simulink model "Abhi"  (R2025a)
settings: Solver=ode45  StartTime=0.0  StopTime=1  RelTol=1e-3  EnableMultiTasking=on
values from neighbouring files (symbols this model uses):
  Bf = 0.001    [Moedl.m]    (also in srm_mpc_setup.m)
  Bp1_Current = linspace(0,180,181)    [Lut.m]    (also in Lut_1.m; Lut_Model.m)
  Bp2_Current = linspace(0,0.50,101)    [Lut.m]    (also in Lut_1.m = linspace(0,10,101); Lut_Model.m = linspace(0,10,101))
  J = 0.01    [CODE.m]    (also in Controller.m = 0.001; Lut.m; Moedl.m; srm_mpc_setup.m)
  LuT_Current = zeros(length(Bp1_Current), length(Bp2_Current))    [Lut.m]    (also in Lut_1.m; Lut_Model.m = zeros(181,101))
  Rs = 1    [CODE.m]    (also in Moedl.m; srm_mpc_setup.m)
undefined symbols (not defined in the file or in its folder): Ion, Lithium
libraries: spsDiodeLib x8, spsSeriesRLCBranchLib x8, spsIGBTLib x6, spsVoltageMeasurementLib x5, spsCurrentMeasurementLib x4, spsMosfetLib x3, simulink_need_slupdate x2, simulink x2, spsBatteryLib x1, mpclib x1, sps_lib x1, spspowerguiLib x1
settings Model: Creator=user 1  LastModifiedBy=srima
settings SolverCC: AlgebraicLoopSolver=TrustRegion
settings DataIOCC: LimitDataPoints=on  SaveFormat=Array  SignalLoggingSaveFormat=ModelDataLogs  ReturnWorkspaceOutputs=off
settings OptimizationCC: ExpressionDepthLimit=2147483647.0  LifeSpan=inf
settings DebuggingCC: UnderspecifiedInitializationDetection=Classic  MergeDetectMultiDrivingBlocksExec=none  SolverPrmCheckMsg=warning  FcnCallInpInsideContextMsg=warning  UnconnectedInputMsg=warning  UnconnectedOutputMsg=warning  UnconnectedLineMsg=warning  StateNameClashWarn=warning  SFUnexpectedBacktrackingDiag=warning  SFNoUnconditionalDefaultTransitionDiag=warning  SFExecutionAtInitializationDiag=none  ArithmeticOperatorsInVariantConditions=warning
settings HardwareCC: ProdBitPerPointer=32.0  ProdBitPerSizeT=32.0  ProdBitPerPtrDiffT=32.0  ProdLargestAtomicFloat=None  ProdIntDivRoundTo=Undefined  ProdEndianess=Unspecified  ProdWordSize=32.0  ProdHWDeviceType=32-bit Generic
settings ModelReferenceCC: PropagateSignalLabelsOutOfModel=off
settings SFSimCC: SimUseLocalCustomCode=off  CustomCodeUndefinedFunction=UseInterfaceOnly
settings RTWCC: RTWUseLocalCustomCode=off  GPUComputeCapability=3.5
settings CodeAppCC: StateflowObjectComments=on
settings GRTTargetCC: TargetLangStandard=C89/C90 (ANSI)  CombineOutputUpdateFcns=off  GRTInterface=on
settings ConfigComp: CovMetricSettings=dw  CovSaveCumulativeToWorkspaceVar=on  CovSaveSingleToWorkspaceVar=on  CovExternalEMLEnable=off
settings SimscapeCC: SimscapeNormalizeSystem=off
settings ConfigurationSet: Description=SimMechanics 2G

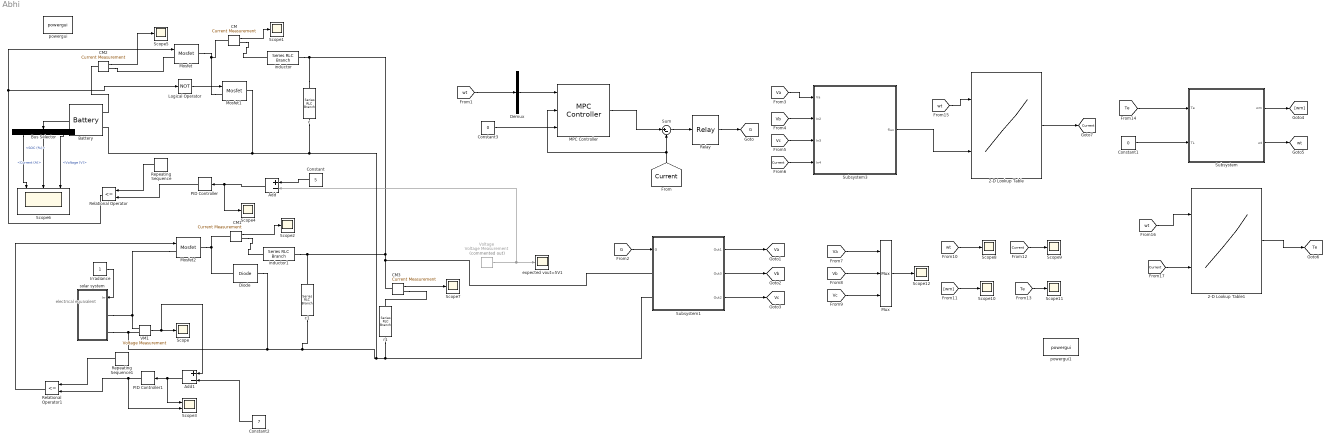
== system Abhi ==
  note: electrical
      | equivalent
  2-D Lookup Table : Lookup_n-D  BreakpointsForDimension1=Bp1_Current  BreakpointsForDimension2=Bp2_Current  Table=LuT_Current  InternalRulePriority=Speed  RndMeth=Simplest
      settings: InputPortMap=u0,u1
  2-D Lookup Table1 : Lookup_n-D  BreakpointsForDimension1=Bp1_Current  BreakpointsForDimension2=Bp2_Current  Table=LuT_Current  InternalRulePriority=Speed  RndMeth=Simplest
      settings: InputPortMap=u0,u1
  Add : Sum  Inputs=+-
  Add1 : Sum  Inputs=+-
  Battery : spsBatteryLib/Battery  BatType=Lithium-Ion  NomV=12  NomQ=6.5  SOC=50  Batt_Tr=30  PresetModel=on  MaxQ=6.5  MinV=9  FullV=13.9678  Dis_rate=2.8261  R=0.018462  Normal_OP=5.8783  expZone="[12.9646     0.319348]"
      settings: LibrarySourceBlock=electricdrivelib/Extra Sources/Battery
  Bus Selector : BusSelector  OutputSignals=SOC (%),Current (A),Voltage (V)
  CM{,1..3} (4 alike) : spsCurrentMeasurementLib/Current Measurement  PhasorSimulation=off  OutputType=Complex  PSBequivalent=0
  Constant : Constant  Value=5
  Constant1 : Constant  Value=0
  Constant2 : Constant  Value=7
  Constant3 : Constant  Value=0
  Demux : Demux  Outputs=3
  Diode : spsDiodeLib/Diode  Ron=0.001  Lon=0  Vf=0.8  IC=0  UseSnubber=off  Rs=500  Cs=250e-9  Measurements=off
  Irradiance : Constant
  Logical Operator : Logic  Operator=NOT  AllPortsSameDT=off  OutDataTypeStr=boolean
  MPC Controller : mpclib/MPC Controller  SCDEnableBlockLinearizationSpecification=on  mpcobj=mpcobj  is_multiple=0  enable_value=0  return_u0=off  updateMPCinCallerWorkspace=on  md_inport=on  mv_inport=off  uref_inport=off  return_cost=off  return_mvseq=off  return_qpstatus=off  return_xseq=off  return_state=off  return_ovseq=off  state_inport=off  umin_inport=off  umax_inport=off  ymin_inport=off  ymax_inport=off  cc_inport=off  ywt_inport=off  uwt_inport=off  duwt_inport=off  rhoeps_inport=off  pm_inport=off  MaximumP=10  HorizonChoice=FixedHorizon  n_ts=0.001  n_p=10  n_mv=1  n_md=1  n_ud=0  n_mo=1  n_uo=0  BlockDataType=double  SampleTimeInherited=off  switch_inport=off
  Mosfet : spsMosfetLib/Mosfet  Ron=0.1  Lon=0  Rd=0.01  Vfd=0  IC=0  Rs=1e5  Cs=inf  Measurements=off
  Mosfet1 : spsMosfetLib/Mosfet  Ron=0.1  Lon=0  Rd=0.01  Vfd=0  IC=0  Rs=1e5  Cs=inf  Measurements=off
  Mosfet2 : spsMosfetLib/Mosfet  Ron=0.1  Lon=0  Rd=0.01  Vfd=0  IC=0  Rs=1e5  Cs=inf  Measurements=off
  Mux : Mux  Inputs=3
  PID Controller : simulink_need_slupdate/PID Controller  P=1  I=5  D=0
  PID Controller1 : simulink_need_slupdate/PID Controller  P=1  I=5  D=0
  Relational Operator : RelationalOperator  Operator=<=  OutDataTypeStr=boolean  InputSameDT=off
  Relational Operator1 : RelationalOperator  Operator=<=  OutDataTypeStr=boolean  InputSameDT=off
  Relay : Relay  OnSwitchValue=10  OffSwitchValue=-10
  Repeating Sequence : simulink/Sources/Repeating Sequence  rep_seq_t=[0 .5/15e3 1/15e3]  rep_seq_y=[0 1 0]
  Repeating Sequence1 : simulink/Sources/Repeating Sequence  rep_seq_t=[0 .5/15e3 1/15e3]  rep_seq_y=[0 1 0]
  Scope{,1..2,4..5,7..12} (11 alike) : Scope
      Scope settings: DataLoggingDecimation=1000  DataLoggingVariableName=pvv  DataLoggingSaveFormat=Array
      Scope1 settings: ActiveDisplayYMinimum=0.5751  ActiveDisplayYMaximum=0.576  DataLoggingDecimation=1000  DataLoggingVariableName=xxbat  DataLoggingSaveFormat=Array
      Scope10 settings: ActiveDisplayYMinimum=-476.34813632584394  ActiveDisplayYMaximum=729.585973445895  DataLoggingVariableName=ScopeData2
      Scope11 settings: ActiveDisplayYMinimum=-0.1626541818945092  ActiveDisplayYMaximum=1.1678030879482377  DataLoggingVariableName=ScopeData5
      Scope12 settings: ActiveDisplayYMinimum=-1  ActiveDisplayYMaximum=1  DataLoggingVariableName=ScopeData6
      Scope2 settings: ActiveDisplayYMinimum=0.5751  ActiveDisplayYMaximum=0.576  DataLoggingDecimation=1000  DataLoggingVariableName=xxpv  DataLoggingSaveFormat=Array
      Scope4 settings: ActiveDisplayYMinimum=-0.7  ActiveDisplayYMaximum=0.5  DataLoggingVariableName=ScopeData3
      Scope5 settings: ActiveDisplayYMinimum=0.5751  ActiveDisplayYMaximum=0.576
      Scope7 settings: ActiveDisplayYMinimum=0.5751  ActiveDisplayYMaximum=0.576  DataLoggingDecimation=1000  DataLoggingVariableName=ioutt  DataLoggingSaveFormat=Array
      Scope8 settings: ActiveDisplayYMinimum=-31.606367633702448  ActiveDisplayYMaximum=124.63641119185642  DataLoggingVariableName=ScopeData8
      Scope9 settings: ActiveDisplayYMinimum=-16.407831336073173  ActiveDisplayYMaximum=26.585137451744139
  Scope3 : Scope  NumInputPorts=2
      settings: ActiveDisplayYMinimum=0.5751  ActiveDisplayYMaximum=0.576  DataLoggingVariableName=ScopeData4
  Scope6 : Scope  NumInputPorts=3
      settings: ActiveDisplayYMinimum=47.5013  ActiveDisplayYMaximum=52.5015  DataLoggingVariableName=ScopeData7
  Subsystem : Subsystem
  Subsystem1 : Subsystem
  Subsystem3 : Subsystem
  Sum : Sum  Inputs=|+-
  VM1 : spsVoltageMeasurementLib/Voltage Measurement  PhasorSimulation=off  OutputType=Complex  PSBequivalent=0
  Voltage : spsVoltageMeasurementLib/Voltage Measurement  Commented=on  PhasorSimulation=off  OutputType=Complex  PSBequivalent=0
  c : spsSeriesRLCBranchLib/Series RLC Branch  LConnTagsString=__new0  RConnTagsString=__new0  BranchType=C  Resistance=1  Inductance=1e-3  SetiL0=off  InitialCurrent=0  Capacitance=160e-6  Setx0=off  InitialVoltage=0  Measurements=None
  c1 : spsSeriesRLCBranchLib/Series RLC Branch  LConnTagsString=__new0  RConnTagsString=__new0  BranchType=C  Resistance=1  Inductance=1e-3  SetiL0=off  InitialCurrent=0  Capacitance=160e-6  Setx0=off  InitialVoltage=0  Measurements=None
  expected vout=5V1 : Scope
      settings: ActiveDisplayYMinimum=-39.820952671630252  ActiveDisplayYMaximum=59.233811839167949  DataLoggingDecimation=1000  DataLoggingVariableName=Vvvv  DataLoggingSaveFormat=Array
  inductor : spsSeriesRLCBranchLib/Series RLC Branch  LConnTagsString=__new0  RConnTagsString=__new0  BranchType=L  Resistance=1  Inductance=3e-3  SetiL0=off  InitialCurrent=0  Capacitance=1e-6  Setx0=off  InitialVoltage=0  Measurements=None
  inductor1 : spsSeriesRLCBranchLib/Series RLC Branch  LConnTagsString=__new0  RConnTagsString=__new0  BranchType=L  Resistance=1  Inductance=3e-3  SetiL0=off  InitialCurrent=0  Capacitance=1e-6  Setx0=off  InitialVoltage=0  Measurements=None
  powergui : sps_lib/powergui  Priority=1  SimulationMode=Discrete  SampleTime=1e-6  frequency=1  Iterations=50  frequencyindice=0  Pbase=100e6  ErrMax=1e-4  UnitsV=kV  UnitsW=MW  buscounter=0  FunctionMessages=off  echomessages=off  EnableUseOfTLC=off  CurrentSourceSwitches=off  DisableSnubberDevices=off  DisableRonSwitches=off  DisableVfSwitches=off  DisplayEquations=off  AutomaticDiscreteSolvers=off  SolverType=Tustin/Backward Euler (TBE)  Interpol=off  ExternalGateDelay=off  methode=off  Ts=100  x0status=blocks  SPID=off  SwTol=0  HookPort=off  NonlinearTolerance=1e-4  nMaxIteration=100  ContinueOnMaxIteration=off  RestoreLinks=warning  ResistiveCurrentMeasurement=off  Frange=[0:2:500]  Ylog=off  Xlog=on  ShowGrid=off  save=off  variable=ZData  structure=0  ZoomFFT=off  StartTime=0.0  cycles=1  DisplayStyle=1  fundamental=60  FreqAxis=off  MaxFrequency=1000  frequencyindicesteady=1  RmsSteady=1  display=off
  powergui1 : spspowerguiLib/powergui  Priority=1  SimulationMode=Discrete  SampleTime=1e-06  frequency=60  Iterations=50  frequencyindice=0  Pbase=100e6  ErrMax=1e-4  UnitsV=kV  UnitsW=MW  buscounter=0  FunctionMessages=off  echomessages=off  EnableUseOfTLC=off  CurrentSourceSwitches=off  DisableSnubberDevices=off  DisableRonSwitches=off  DisableVfSwitches=off  DisplayEquations=off  AutomaticDiscreteSolvers=off  SolverType=Tustin/Backward Euler (TBE)  Interpol=off  ExternalGateDelay=off  methode=off  Ts=100  x0status=blocks  SPID=on  SwTol=0  HookPort=off  NonlinearTolerance=1e-4  nMaxIteration=100  ContinueOnMaxIteration=off  RestoreLinks=warning  ResistiveCurrentMeasurement=off  Frange=[0:2:500]  Ylog=off  Xlog=on  ShowGrid=off  save=off  variable=ZData  structure=0  ZoomFFT=off  StartTime=0.0  cycles=1  DisplayStyle=1  fundamental=60  FreqAxis=off  MaxFrequency=1000  frequencyindicesteady=1  RmsSteady=1  display=off
  r1 : spsSeriesRLCBranchLib/Series RLC Branch  LConnTagsString=__new0  RConnTagsString=__new0  BranchType=R  Resistance=75  Inductance=1e-3  SetiL0=off  InitialCurrent=0  Capacitance=1e-6  Setx0=off  InitialVoltage=0  Measurements=None
  solar system : Subsystem
  tag scope: Current=global, G=global, Te=global, Va=global, Vb=global, Vc=global, wt=global
  wires:
  Add/1 -> PID Controller/1, Scope4/1
  Repeating Sequence/1 -> Relational Operator/1
  Constant/1 -> Add/1
  CM/1 -> Scope1/1
  PID Controller/1 -> Relational Operator/2
  Relational Operator/1 -> Mosfet/1, Logical Operator/1
  Add1/1 -> PID Controller1/1, Scope3/1
  Repeating Sequence1/1 -> Relational Operator1/1
  Voltage/1 -> expected vout=5V1/1, Add/2
  CM1/1 -> Scope2/1
  PID Controller1/1 -> Relational Operator1/2, Scope3/2
  Relational Operator1/1 -> Mosfet2/1
  Constant2/1 -> Add1/2
  Irradiance/1 -> solar system/1(Irr)
  VM1/1 -> Scope/1, Add1/1
  Logical Operator/1 -> Mosfet1/1
  CM2/1 -> Scope5/1
  Battery/1 -> Bus Selector/1
  Bus Selector/3 -> Scope6/3  "<Voltage (V)>"
  Bus Selector/2 -> Scope6/2  "<Current (A)>"
  Bus Selector/1 -> Scope6/1  "<SOC (%)>"
  CM3/1 -> Scope7/1
  Constant1/1 -> Subsystem/2(TL)
  [wt] -> 2-D Lookup Table1/1
  Subsystem1/1(Out1) -> [Va]
  [Vc] -> Subsystem3/3(In3)
  [Current] -> Scope9/1
  Sum/1 -> Relay/1
  [wm] -> Scope10/1
  [wt] -> Scope8/1
  Subsystem1/2(Out3) -> [Vb]
  [wt] -> 2-D Lookup Table/1
  2-D Lookup Table1/1 -> [Te]
  [Current] -> 2-D Lookup Table1/2
  2-D Lookup Table/1 -> [Current]
  [G] -> Subsystem1/1(G)
  [Te] -> Scope11/1
  [Va] -> Subsystem3/1(Va)
  [Vb] -> Subsystem3/2(In2)
  [wt] -> Demux/1
  [Va] -> Mux/1
  Relay/1 -> [G]
  [Current] -> Sum/2, MPC Controller/2
  [Te] -> Subsystem/1(Te)
  Subsystem/1(wm) -> [wm]
  Mux/1 -> Scope12/1
  [Current] -> Subsystem3/4(In4)
  Subsystem/2(wt) -> [wt]
  [Vc] -> Mux/3
  [Vb] -> Mux/2
  Subsystem3/1(flux) -> 2-D Lookup Table/2
  Subsystem1/3(Out2) -> [Vc]
  MPC Controller/1 -> Sum/1
  Constant3/1 -> MPC Controller/3
  Demux/2 -> MPC Controller/1
  connections:
  Mosfet1/LConn1 -- Mosfet/RConn1 -- CM/LConn1
  Mosfet2/RConn1 -- Diode/RConn1 -- CM1/LConn1
  c/LConn1 -- inductor/RConn1 -- Subsystem1/LConn1 -- CM3/LConn1 -- inductor1/RConn1 -- c1/LConn1
  Mosfet2/LConn1 -- solar system/LConn1 -- VM1/LConn1
  CM2/RConn1 -- Mosfet/LConn1
  CM/RConn1 -- inductor/LConn1
  CM1/RConn1 -- inductor1/LConn1
  CM2/LConn1 -- Battery/LConn1
  CM3/RConn1 -- r1/LConn1
  Battery/LConn2 -- Mosfet1/RConn1 -- c/RConn1 -- c1/RConn1 -- solar system/LConn2 -- VM1/LConn2 -- Diode/LConn1 -- Subsystem1/LConn2 -- r1/RConn1

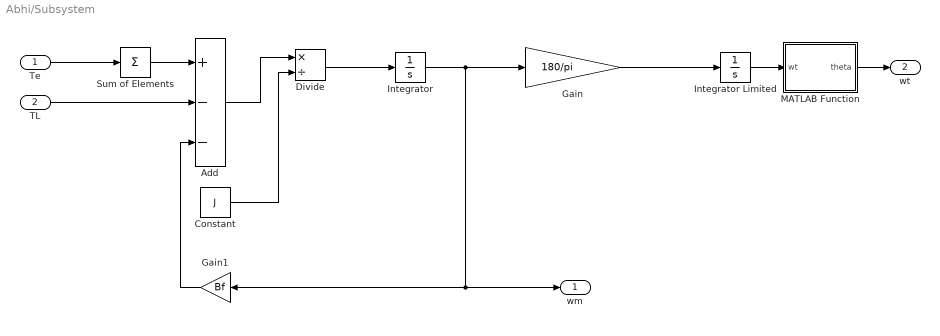
== system Abhi/Subsystem ==
  Te : Inport
  TL : Inport  Port=2
  Add : Sum  Inputs=+--
  Constant : Constant  Value=J
  Divide : Product  Inputs=*/
  Gain : Gain  Gain=180/pi
  Gain1 : Gain  Gain=Bf
  Integrator : Integrator
  Integrator Limited : Integrator  InitialCondition=[0,30,60]  LimitOutput=on
  MATLAB Function : MATLAB Function  TreatAsAtomicUnit=on
  Sum of Elements : Sum  Inputs=+
  wm : Outport
  wt : Outport  Port=2
  wires:
  Te/1 -> Sum of Elements/1
  Sum of Elements/1 -> Add/1
  TL/1 -> Add/2
  Gain1/1 -> Add/3
  Divide/1 -> Integrator/1
  Add/1 -> Divide/1
  Constant/1 -> Divide/2
  Gain/1 -> Integrator Limited/1
  Integrator/1 -> wm/1, Gain1/1, Gain/1
  MATLAB Function/1(theta) -> wt/1
  Integrator Limited/1 -> MATLAB Function/1(wt)

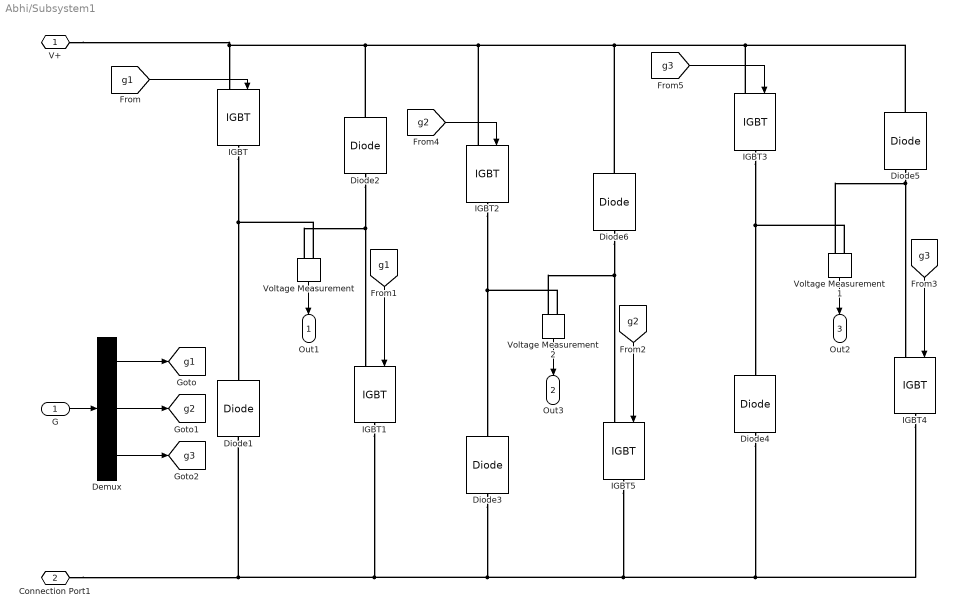
== system Abhi/Subsystem1 ==
  G : Inport
  Demux : Demux  Outputs=3
  Diode1 : spsDiodeLib/Diode  Ron=1e-3  Lon=0  Vf=0.8  IC=0  UseSnubber=0  Rs=1000  Cs=inf  Measurements=off
  Diode2 : spsDiodeLib/Diode  Ron=0.001  Lon=0  Vf=0.8  IC=0  UseSnubber=0  Rs=500  Cs=250e-9  Measurements=off
  Diode3 : spsDiodeLib/Diode  Ron=1e-3  Lon=0  Vf=0.8  IC=0  UseSnubber=0  Rs=1000  Cs=inf  Measurements=off
  Diode4 : spsDiodeLib/Diode  Ron=1e-3  Lon=0  Vf=0.8  IC=0  UseSnubber=0  Rs=1000  Cs=inf  Measurements=off
  Diode5 : spsDiodeLib/Diode  Ron=0.001  Lon=0  Vf=0.8  IC=0  UseSnubber=0  Rs=500  Cs=250e-9  Measurements=off
  Diode6 : spsDiodeLib/Diode  Ron=0.001  Lon=0  Vf=0.8  IC=0  UseSnubber=0  Rs=500  Cs=250e-9  Measurements=off
  IGBT{,1..5} (6 alike) : spsIGBTLib/IGBT  Ron=0.001  Lon=0  Vf=1  Tf=1e-6  Tt=2e-6  IC=0  Rs=1e5  Cs=inf  Measurements=off
  Voltage Measurement : spsVoltageMeasurementLib/Voltage Measurement  PhasorSimulation=off  OutputType=Complex  PSBequivalent=0
  Voltage Measurement1 : spsVoltageMeasurementLib/Voltage Measurement  PhasorSimulation=off  OutputType=Complex  PSBequivalent=0
  Voltage Measurement2 : spsVoltageMeasurementLib/Voltage Measurement  PhasorSimulation=off  OutputType=Complex  PSBequivalent=0
  V+ : PMIOPort  Side=Left
  Connection Port1 : PMIOPort  Port=2  Side=Left
  Out1 : Outport
  Out3 : Outport  Port=2
  Out2 : Outport  Port=3
  tag scope: g1=global, g2=global, g3=global
  wires:
  G/1 -> Demux/1
  Demux/1 -> [g1]
  Demux/3 -> [g3]
  Demux/2 -> [g2]
  [g1] -> IGBT/1
  [g1] -> IGBT1/1
  Voltage Measurement/1 -> Out1/1
  Voltage Measurement1/1 -> Out2/1
  [g3] -> IGBT4/1
  [g2] -> IGBT5/1
  Voltage Measurement2/1 -> Out3/1
  [g2] -> IGBT2/1
  [g3] -> IGBT3/1
  connections:
  V+/RConn1 -- Diode5/RConn1 -- IGBT3/LConn1 -- Diode6/RConn1 -- IGBT2/LConn1 -- Diode2/RConn1 -- IGBT/LConn1
  IGBT/RConn1 -- Voltage Measurement/LConn1 -- Diode1/RConn1
  Connection Port1/RConn1 -- IGBT4/RConn1 -- Diode4/LConn1 -- IGBT5/RConn1 -- Diode3/LConn1 -- IGBT1/RConn1 -- Diode1/LConn1
  Diode2/LConn1 -- Voltage Measurement/LConn2 -- IGBT1/LConn1
  Diode5/LConn1 -- Voltage Measurement1/LConn2 -- IGBT4/LConn1
  IGBT3/RConn1 -- Voltage Measurement1/LConn1 -- Diode4/RConn1
  IGBT2/RConn1 -- Voltage Measurement2/LConn1 -- Diode3/RConn1
  Diode6/LConn1 -- Voltage Measurement2/LConn2 -- IGBT5/LConn1

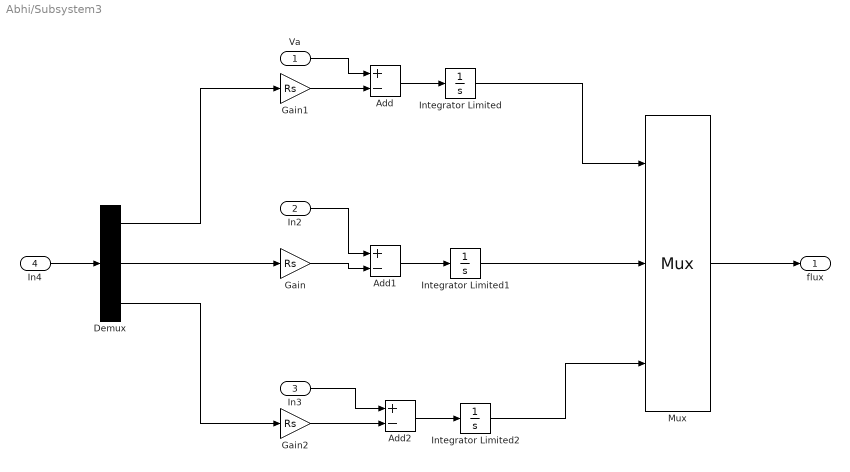
== system Abhi/Subsystem3 ==
  Va : Inport
  In2 : Inport  Port=2
  In3 : Inport  Port=3
  In4 : Inport  Port=4
  Add : Sum  Inputs=+-
  Add1 : Sum  Inputs=+-
  Add2 : Sum  Inputs=+-
  Demux : Demux  Outputs=3
  Gain : Gain  Gain=Rs
  Gain1 : Gain  Gain=Rs
  Gain2 : Gain  Gain=Rs
  Integrator Limited : Integrator  LimitOutput=on  UpperSaturationLimit=1  LowerSaturationLimit=0
  Integrator Limited1 : Integrator  LimitOutput=on  UpperSaturationLimit=1  LowerSaturationLimit=0
  Integrator Limited2 : Integrator  LimitOutput=on  UpperSaturationLimit=1  LowerSaturationLimit=0
  Mux : Mux  Inputs=3
  flux : Outport
  wires:
  In4/1 -> Demux/1
  Demux/1 -> Gain1/1
  Demux/2 -> Gain/1
  Demux/3 -> Gain2/1
  In3/1 -> Add2/1
  Gain2/1 -> Add2/2
  In2/1 -> Add1/1
  Gain/1 -> Add1/2
  Gain1/1 -> Add/2
  Va/1 -> Add/1
  Add2/1 -> Integrator Limited2/1
  Add1/1 -> Integrator Limited1/1
  Add/1 -> Integrator Limited/1
  Integrator Limited/1 -> Mux/1
  Integrator Limited1/1 -> Mux/2
  Integrator Limited2/1 -> Mux/3
  Mux/1 -> flux/1

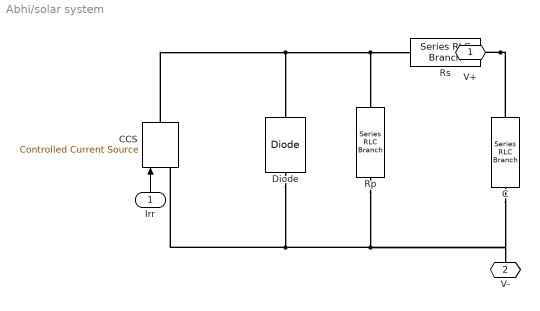
== system Abhi/solar system ==
  Irr : Inport
  C : spsSeriesRLCBranchLib/Series RLC Branch  LConnTagsString=__new0  RConnTagsString=__new0  BranchType=C  Resistance=0.1  Inductance=1e-3  SetiL0=off  InitialCurrent=0  Capacitance=100e-6  Setx0=off  InitialVoltage=0  Measurements=None
  CCS : spsControlledCurrentSourceLib/Controlled Current Source  Initialize=on  Source_Type=DC  Amplitude=0  Phase=0  Frequency=0  Measurements=None
  Diode : spsDiodeLib/Diode  Ron=0.001  Lon=0  Vf=8.75  IC=0  UseSnubber=off  Rs=500  Cs=250e-9  Measurements=off
  Rp : spsSeriesRLCBranchLib/Series RLC Branch  LConnTagsString=__new0  RConnTagsString=__new0  BranchType=R  Resistance=10000  Inductance=1e-3  SetiL0=off  InitialCurrent=0  Capacitance=1e-6  Setx0=off  InitialVoltage=0  Measurements=None
  Rs : spsSeriesRLCBranchLib/Series RLC Branch  LConnTagsString=__new0  RConnTagsString=__new0  BranchType=R  Resistance=0.1  Inductance=1e-3  SetiL0=off  InitialCurrent=0  Capacitance=1e-6  Setx0=off  InitialVoltage=0  Measurements=None
  V+ : PMIOPort  Side=Left
  V- : PMIOPort  Port=2  Side=Left
  wires:
  Irr/1 -> CCS/1
  connections:
  C/LConn1 -- V+/RConn1 -- Rs/RConn1
  Diode/RConn1 -- Rp/RConn1 -- C/RConn1 -- V-/RConn1 -- CCS/LConn1
  CCS/RConn1 -- Diode/LConn1 -- Rs/LConn1 -- Rp/LConn1

== matlab function Abhi/Subsystem/MATLAB Function ==
  data: wt input; theta output
function theta = fcn(wt)

theta = mod(wt,90);
